simulink model "sim_model"  (Simulink 8.0)
settings: Solver=ode45  StartTime=0.0  StopTime=20  RelTol=1e-3
libraries: fmu_me_lib x1
settings Model: Creator=Tin Rabuzin  LastModifiedBy=Tin Rabuzin
settings DebuggingCC: SolverPrmCheckMsg=none

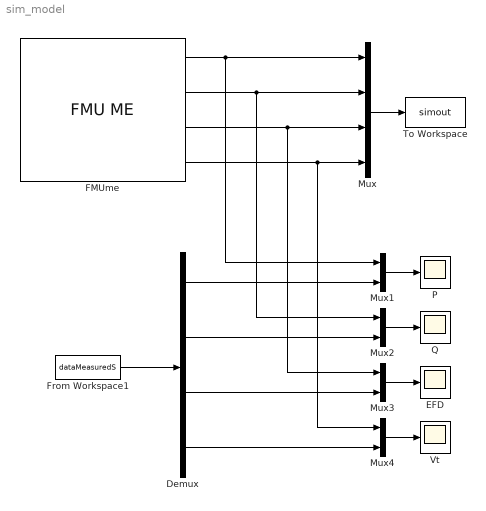
== system sim_model ==
  Demux : Demux
  EFD : Scope
      settings: YMin=0.5  YMax=5.5  SaveName=ScopeData2
  FMUme : fmu_me_lib/FMU ME  Description=Simulates an FMU for Model Exchange 1.0 or Model Exchange 2.0.
  From Workspace1 : FromWorkspace  VariableName=dataMeasuredS  SampleTime=0
  Mux : Mux
  Mux{1..4} (4 alike) : Mux  Inputs=2
  P : Scope
      settings: YMin=0.155  YMax=0.1925
  Q : Scope
      settings: YMin=-0.15  YMax=0.55
  To Workspace : ToWorkspace  VariableName=simout  SampleTime=-1  SaveFormat=Structure With Time
  Vt : Scope
      settings: YMin=0.96  YMax=1.025  SaveName=ScopeData3
  wires:
  Mux/1 -> To Workspace/1
  From Workspace1/1 -> Demux/1
  Mux1/1 -> P/1
  Mux2/1 -> Q/1
  Mux3/1 -> EFD/1
  Mux4/1 -> Vt/1
  FMUme/1 -> Mux1/1, Mux/1
  FMUme/2 -> Mux2/1, Mux/2
  FMUme/3 -> Mux3/1, Mux/3
  FMUme/4 -> Mux4/1, Mux/4
  Demux/1 -> Mux1/2
  Demux/2 -> Mux2/2
  Demux/3 -> Mux3/2
  Demux/4 -> Mux4/2
